simulink model "DiagramaDCcampo"  (R2017b)
settings: Solver=VariableStepAuto  StartTime=0.0  StopTime=10.0  RelTol=1e-3
values from neighbouring files (symbols this model uses):
  B = 0.002953    [Graficas.m]
  J = 0.0221    [Graficas.m]
  Kt = 0.516    [Graficas.m]
  Lf = 156    [Graficas.m]
  Rf = 281.3    [Graficas.m]
  ST = 1    [Graficas.m]
  Td = 0    [Graficas.m]
  VF = 240    [Graficas.m]
  VI = 140    [Graficas.m]
settings Model: Creator=usuario  LastModifiedBy=Wilmer
settings SFSimCC: SimUseLocalCustomCode=on
settings RTWCC: RTWUseLocalCustomCode=on
settings CodeAppCC: StateflowObjectComments=on

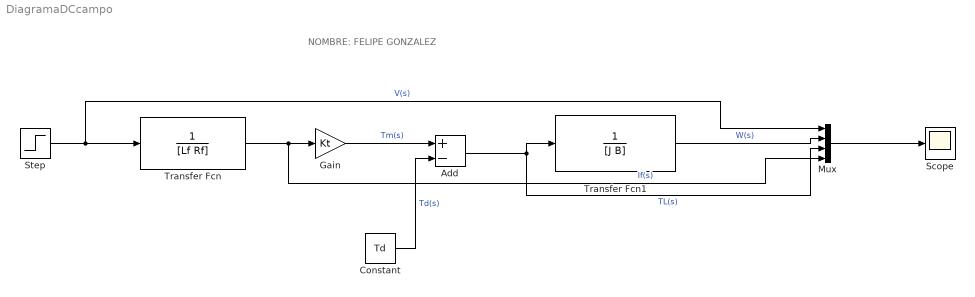
== system DiagramaDCcampo ==
  note: NOMBRE: FELIPE GONZALEZ
  Add : Sum  Inputs=+-
  Constant : Constant  Value=Td
  Gain : Gain  Gain=Kt
  Mux : Mux
  Scope : Scope
  Step : Step  Time=ST  Before=VI  After=VF  SampleTime=0
  Transfer Fcn : TransferFcn  Denominator=[Lf Rf]
  Transfer Fcn1 : TransferFcn  Denominator=[J B]
  wires:
  Gain/1 -> Add/1  "Tm(s)"
  Constant/1 -> Add/2  "Td(s)"
  Add/1 -> Mux/3, Transfer Fcn1/1  "TL(s)"
  Transfer Fcn1/1 -> Mux/2  "W(s)"
  Mux/1 -> Scope/1
  Step/1 -> Mux/1, Transfer Fcn/1  "V(s)"
  Transfer Fcn/1 -> Mux/4, Gain/1  "If(s)"
